simulink model "Doppelpendel"  (R2015b)
settings: Solver=ode4  StartTime=0.0  StopTime=60.0  FixedStep=0.001  RelTol=1e-3
PreLoadFcn:
  | l_1 = 0.194;
  | l_2 = 0.1855;
  | m_w = 0.8101;
  | m_1 = 0.0313;
  | m_2 = 0.0313;
  | m_3 = 0.0308;
  | dp_1 = 0.00045; %0.001;
  | dp_2 = 0.00045;
  | d_m = 0.0005;
  | r = 0.011935;
  | J_Motor = 0.0000462;
InitFcn:
  | Rueckfuervektor_Beobachter_Doppelpendel
values from neighbouring files (symbols this model uses):
  Ad = expm(A*T)    [Rueckfuervektor_Beobachter_Doppelpendel.m]
  Bd = integral(fun,0,T,'ArrayValued',true)    [Rueckfuervektor_Beobachter_Doppelpendel.m]
  C = [ 1 , 0 , 0 , 0 ]    [Rueckfuervektor_Beobachter_Doppelpendel.m]
  g = 9.81    [Rueckfuervektor_Beobachter_Doppelpendel.m]
  Hd = place(Ad',C',pd).'    [Rueckfuervektor_Beobachter_Doppelpendel.m]
  K_6 = place(A_6,B_6,p_6)    [Rueckfuervektor_Beobachter_Doppelpendel.m]
  T = 0.001    [Rueckfuervektor_Beobachter_Doppelpendel.m]
libraries: simulink x3
settings Model: Creator=behm  LastModifiedBy=serov
settings DataIOCC: SaveFormat=Array
settings DebuggingCC: SolverPrmCheckMsg=warning
settings HardwareCC: ProdBitPerPointer=32  ProdLargestAtomicFloat=None  ProdIntDivRoundTo=Undefined  ProdEndianess=Unspecified  ProdWordSize=32  ProdHWDeviceType=32-bit Generic
settings GRTTargetCC: GeneratePreprocessorConditionals=Disable all
settings ConfigComp: CovModelRefEnable=Off  CovSFcnEnable=off

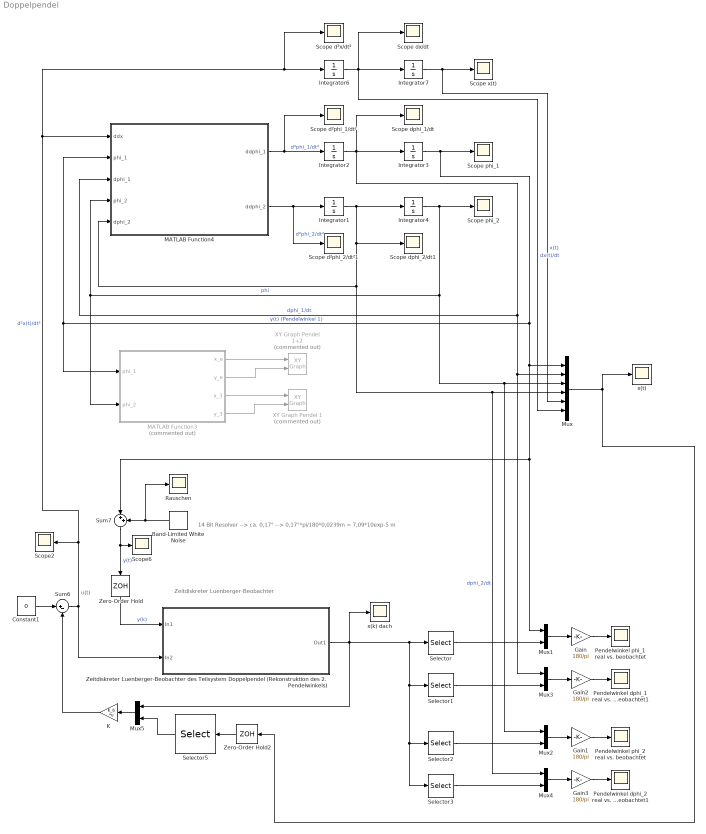
== system Doppelpendel ==
  note: u(t)
  note: 14 Bit Resolver --> ca. 0,17° --> 0,17°*pi/180*0,0239m = 7,09*10exp-5 m
  note: Zeitdiskreter Luenberger-Beobachter
  Band-Limited White Noise : simulink/Sources/Band-Limited White Noise  Cov=0.5*0.000000003  Ts=0.001  seed=[23341]
  Constant1 : Constant  Value=0
  Gain{,1..3} (4 alike) : Gain  Gain=180/pi
  Integrator{1..3,6..7} (5 alike) : Integrator
  Integrator4 : Integrator  InitialCondition=0.0174
  K : Gain  Gain=K_6  Multiplication=Matrix(K*u) (u vector)  SampleTime=T
  MATLAB Function3 : MATLAB Function  Commented=on  TreatAsAtomicUnit=on
  MATLAB Function4 : MATLAB Function  TreatAsAtomicUnit=on
  Mux : Mux  Inputs=6
  Mux{1..5} (5 alike) : Mux  Inputs=2
  Pendelwinkel dphi_1 real vs. beobachtet1 : Scope
  Pendelwinkel dphi_2 real vs. beobachtet1 : Scope
  Pendelwinkel phi_1 real vs. beobachtet : Scope
  Pendelwinkel phi_2 real vs. beobachtet : Scope
  Rauschen : Scope
  Scope dphi_1/dt : Scope
  Scope dphi_2/dt1 : Scope
  Scope dx/dt : Scope
  Scope d²phi_1/dt² : Scope
  Scope d²phi_2/dt²1 : Scope
  Scope d²x/dt² : Scope
  Scope phi_1 : Scope
  Scope phi_2 : Scope
  Scope x(t) : Scope
  Scope2 : Scope
  Scope6 : Scope
  Selector : Selector  InputPortWidth=4  IndexOptions=Index vector (dialog)  Indices=[1]  OutputSizes=1
  Selector1 : Selector  InputPortWidth=4  IndexOptions=Index vector (dialog)  Indices=[2]  OutputSizes=1
  Selector2 : Selector  InputPortWidth=4  IndexOptions=Index vector (dialog)  Indices=[3]  OutputSizes=1
  Selector3 : Selector  InputPortWidth=4  IndexOptions=Index vector (dialog)  Indices=[4]  OutputSizes=1
  Selector5 : Selector  InputPortWidth=6  IndexOptions=Index vector (dialog)  Indices=[5 6]  OutputSizes=1
  Sum6 : Sum  Inputs=|+-  SampleTime=T
  Sum7 : Sum  Inputs=|++
  XY Graph Pendel 1 : simulink/Sinks/XY Graph  Commented=on  xmin=-0.7  xmax=0.7  ymin=0  ymax=0.7  st=-1
  XY Graph Pendel 1+2 : simulink/Sinks/XY Graph  Commented=on  xmin=-0.7  xmax=0.7  ymin=0  ymax=0.7  st=-1
  Zeitdiskreter Luenberger-Beobachter des Teilsystem Doppelpendel (Rekonstruktion des 2. Pendelwinkels) : Subsystem
  Zero-Order Hold : ZeroOrderHold  SampleTime=T
  Zero-Order Hold2 : ZeroOrderHold  SampleTime=T
  x(k) dach : Scope
  x(t) : Scope
  wires:
  Sum6/1 -> Zeitdiskreter Luenberger-Beobachter des Teilsystem Doppelpendel (Rekonstruktion des 2. Pendelwinkels)/2(In2), MATLAB Function4/1(ddx), Scope d²x/dt²/1, Integrator6/1, Scope2/1  "d²x(t)/dt²"
  MATLAB Function4/1(ddphi_1) -> Scope d²phi_1/dt²/1, Integrator2/1  "d²phi_1/dt²"
  Integrator2/1 -> Mux3/1, Mux/2, MATLAB Function4/3(dphi_1), Scope dphi_1/dt/1, Integrator3/1  "dphi_1/dt"
  MATLAB Function4/2(ddphi_2) -> Scope d²phi_2/dt²1/1, Integrator1/1  "d²phi_2/dt²"
  Integrator1/1 -> Mux4/1, Mux/4, MATLAB Function4/5(dphi_2), Scope dphi_2/dt1/1, Integrator4/1  "dphi_2/dt"
  MATLAB Function3/1(x_e) -> XY Graph Pendel 1+2/1
  MATLAB Function3/2(y_e) -> XY Graph Pendel 1+2/2
  MATLAB Function3/3(x_3) -> XY Graph Pendel 1/1
  MATLAB Function3/4(y_3) -> XY Graph Pendel 1/2
  Integrator4/1 -> Mux/3, Mux2/1, MATLAB Function3/2(phi_2), MATLAB Function4/4(phi_2), Scope phi_2/1  "phi"
  Integrator3/1 -> Sum7/1, Mux1/1, Mux/1, MATLAB Function3/1(phi_1), MATLAB Function4/2(phi_1), Scope phi_1/1  "y(t) (Pendelwinkel 1)"
  Sum7/1 -> Zero-Order Hold/1, Scope6/1  "y(t)"
  Band-Limited White Noise/1 -> Sum7/2, Rauschen/1
  Mux1/1 -> Gain/1
  Selector/1 -> Mux1/2
  Constant1/1 -> Sum6/1
  Mux2/1 -> Gain1/1
  Selector2/1 -> Mux2/2
  K/1 -> Sum6/2
  Integrator6/1 -> Scope dx/dt/1, Mux/6, Integrator7/1  "dx(t)/dt"
  Integrator7/1 -> Mux/5, Scope x(t)/1  "x(t)"
  Gain/1 -> Pendelwinkel phi_1 real vs. beobachtet/1
  Gain1/1 -> Pendelwinkel phi_2 real vs. beobachtet/1
  Mux3/1 -> Gain2/1
  Selector1/1 -> Mux3/2
  Mux4/1 -> Gain3/1
  Selector3/1 -> Mux4/2
  Gain2/1 -> Pendelwinkel dphi_1 real vs. beobachtet1/1
  Gain3/1 -> Pendelwinkel dphi_2 real vs. beobachtet1/1
  Mux/1 -> x(t)/1, Zero-Order Hold2/1
  Zero-Order Hold2/1 -> Selector5/1
  Mux5/1 -> K/1
  Selector5/1 -> Mux5/2
  Zeitdiskreter Luenberger-Beobachter des Teilsystem Doppelpendel (Rekonstruktion des 2. Pendelwinkels)/1(Out1) -> Mux5/1, Selector3/1, Selector2/1, Selector1/1, Selector/1, x(k) dach/1
  Zero-Order Hold/1 -> Zeitdiskreter Luenberger-Beobachter des Teilsystem Doppelpendel (Rekonstruktion des 2. Pendelwinkels)/1(In1)  "y(k)"

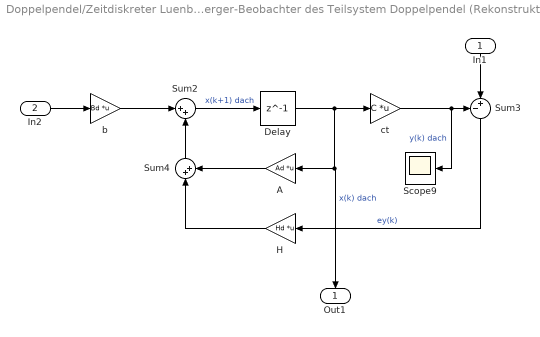
== system Doppelpendel/Zeitdiskreter Luenberger-Beobachter des Teilsystem Doppelpendel (Rekonstruktion des 2. Pendelwinkels) ==
  In1 : Inport
  In2 : Inport  Port=2
  A : Gain  Gain=Ad  Multiplication=Matrix(K*u) (u vector)  SampleTime=T
  Delay : Delay  DelayLength=1  SampleTime=T
  H : Gain  Gain=Hd  Multiplication=Matrix(K*u)  SampleTime=T
  Scope9 : Scope
  Sum2 : Sum  Inputs=|++  SampleTime=T
  Sum3 : Sum  Inputs=-+|  SampleTime=T
  Sum4 : Sum  Inputs=|++  SampleTime=T
  b : Gain  Gain=Bd  Multiplication=Matrix(K*u)  SampleTime=T  LockScale=on
  ct : Gain  Gain=C  Multiplication=Matrix(K*u) (u vector)  SampleTime=T
  Out1 : Outport
  wires:
  H/1 -> Sum4/1
  Sum3/1 -> H/1  "ey(k)"
  ct/1 -> Scope9/1, Sum3/1  "y(k) dach"
  b/1 -> Sum2/1
  A/1 -> Sum4/2
  Sum2/1 -> Delay/1  "x(k+1) dach"
  In1/1 -> Sum3/2
  Sum4/1 -> Sum2/2
  Delay/1 -> Out1/1, A/1, ct/1  "x(k) dach"
  In2/1 -> b/1

== matlab function Doppelpendel/MATLAB Function3 ==
  data: phi_1 input; phi_2 input; l_1 parameter; l_2 parameter; x_e output; y_e output; x_3 output; y_3 output
function [x_e,y_e,x_3,y_3] = Position_der_Pendelspitze(phi_1, phi_2, l_1, l_2)
%#codegen

x_e = - l_1*sin(phi_1) - l_2*sin(phi_2);
y_e =   l_1*cos(phi_1) + l_2*cos(phi_2);

x_3 = - l_1*sin(phi_1);
y_3 =   l_1*cos(phi_1);

== matlab function Doppelpendel/MATLAB Function4 ==
  data: ddx input; phi_1 input; dphi_1 input; phi_2 input; ddphi_1 output; dphi_2 input; ddphi_2 output; l_1 parameter; l_2 parameter; g parameter; m_1 parameter; m_2 parameter; m_3 parameter; dp_1 parameter; dp_2 parameter
function [ddphi_1, ddphi_2] = Doppelpendel(ddx, phi_1, dphi_1, phi_2, dphi_2, l_1, l_2, g, m_1, m_2, m_3, dp_1, dp_2)
%#codegen

J_1 = 1/12*m_1*l_1^2 + 0.00002; %% (um den Schwerpunkt)
J_2 = 1/12*m_2*l_2^2; %% (um den Schwerpunkt)


% ddphi_1 = -2 / ( l_1^2*(m_1+4*m_2+4*m_3+4*J_1) ) * ( l_1*l_2*m_2*sin(phi_2-phi_2)*dphi_2^2 ...
%                                                     + l_1*l_2*m_2*cos(phi_1-phi_2)*ddphi_2 ...
%                                                     - l_1*(m_1+2*m_2+2*m_3)*cos(phi_1)*ddx ...
%                                                     - l_1*(m_1+2*m_2+2*m_3)*g*sin(phi_1) ...
%                                                     + 2*dp_2*(dphi_2-dphi_1) + 2*dp_1*dphi_1 );

ddphi_1 = (9*l_1*(dphi_1^2*l_1*l_2*m_2*sin(phi_1-phi_2)+g*sin(phi_2)*l_2*m_2+cos(phi_2)*l_2*m_2*ddx+2*dp_2*dphi_1-2*dp_2*dphi_2)*cos(phi_1-phi_2)-6*(-dphi_2^2*l_1*l_2*m_2*sin(phi_1-phi_2)+cos(phi_1)*l_1*(m_1+2*m_2+2*m_3)*ddx+(2*dp_2-2*dp_1)*dphi_1-2*dp_2*dphi_2+g*sin(phi_1)*l_1*(m_1+2*m_2+2*m_3))*l_2)/l_1^2/(9*cos(phi_1-phi_2)^2*m_2-12*m_3-12*m_2-4*m_1)/l_2;

ddphi_2 = (9*(-dphi_2^2*l_1*l_2*m_2*sin(phi_1-phi_2)+cos(phi_1)*l_1*(m_1+2*m_2+2*m_3)*ddx+(2*dp_2-2*dp_1)*dphi_1-2*dp_2*dphi_2+g*sin(phi_1)*l_1*(m_1+2*m_2+2*m_3))*m_2*l_2*cos(phi_1-phi_2)-6*l_1*(m_1+3*m_2+3*m_3)*(dphi_1^2*l_1*l_2*m_2*sin(phi_1-phi_2)+g*sin(phi_2)*l_2*m_2+cos(phi_2)*l_2*m_2*ddx+2*dp_2*dphi_1-2*dp_2*dphi_2))/l_2^2/l_1/(9*cos(phi_1-phi_2)^2*m_2-12*m_3-12*m_2-4*m_1)/m_2;
